simulink model "likestromsmotor"  (R2015a)
settings: Solver=ode45  StartTime=0.0  StopTime=10.0  RelTol=1e-3
values from neighbouring files (symbols this model uses):
  J_m = 0.01    [main.m]
  K_e = K_m    (= 1)    [main.m]
  K_m = 1    [main.m]
  L_a = 1    [main.m]
  M_L = 0    [main.m]
  R_a = 10    [main.m]
  theta_r = pi/2    (= 1.57079632679)    [main.m]
libraries: simulink x1
settings Model: Creator=Martin  LastModifiedBy=Martin

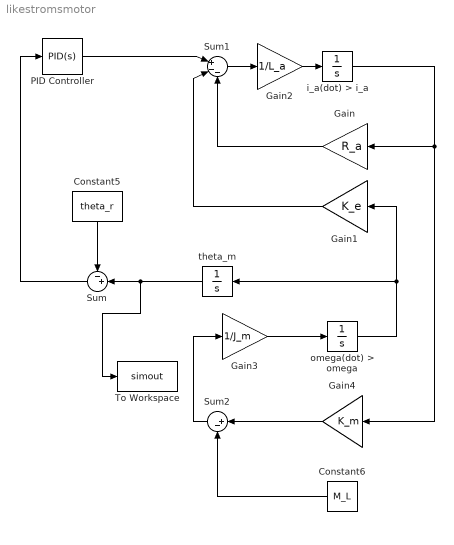
== system likestromsmotor ==
  Constant5 : Constant  Value=theta_r
  Constant6 : Constant  Value=M_L
  Gain : Gain  Gain=R_a
  Gain1 : Gain  Gain=K_e
  Gain2 : Gain  Gain=1/L_a
  Gain3 : Gain  Gain=1/J_m
  Gain4 : Gain  Gain=K_m
  PID Controller : simulink/Continuous/PID Controller  Controller=PID  TimeDomain=Continuous-time  SampleTime=-1  IntegratorMethod=Forward Euler  FilterMethod=Forward Euler  Form=Ideal  UseFilter=on  ControllerParametersSource=internal  P=1  I=0  D=0  N=100  InitialConditionSource=internal  InitialConditionForIntegrator=0  InitialConditionForFilter=0  ExternalReset=none  LimitOutput=off  UpperSaturationLimit=inf  LowerSaturationLimit=-inf  LinearizeAsGain=on  AntiWindupMode=none  Kb=1  TrackingMode=off  Kt=1  PParamMin=[]  PParamMax=[]  IParamMin=[]  IParamMax=[]  DParamMin=[]  DParamMax=[]  NParamMin=[]  NParamMax=[]  KbParamMin=[]  KbParamMax=[]  KtParamMin=[]  KtParamMax=[]  POutMin=[]  POutMax=[]  IOutMin=[]  IOutMax=[]  DOutMin=[]  DOutMax=[]  NOutMin=[]  NOutMax=[]  KbOutMin=[]  KbOutMax=[]  KtOutMin=[]  KtOutMax=[]  IntegratorOutMin=[]  IntegratorOutMax=[]  FilterOutMin=[]  FilterOutMax=[]  SumOutMin=[]  SumOutMax=[]  SumI1OutMin=[]  SumI1OutMax=[]  SumI2OutMin=[]  SumI2OutMax=[]  SumI3OutMin=[]  SumI3OutMax=[]  SumDOutMin=[]  SumDOutMax=[]  SaturationOutMin=[]  SaturationOutMax=[]  IntegratorContinuousStateAttributes=''  IntegratorStateMustResolveToSignalObject=off  IntegratorRTWStateStorageClass=Auto  FilterContinuousStateAttributes=''  FilterStateMustResolveToSignalObject=off  FilterRTWStateStorageClass=Auto  DifferentiatorICPrevScaledInput=0  DifferentiatorOutMin=[]  DifferentiatorOutMax=[]
  Sum : Sum  Inputs=-+|
  Sum1 : Sum  Inputs=|+--
  Sum2 : Sum  Inputs=|+-
  To Workspace : ToWorkspace  VariableName=simout  SaveFormat=Timeseries  SampleTime=-1
  i_a(dot) > i_a : Integrator
  omega(dot) > omega : Integrator
  theta_m : Integrator
  wires:
  Constant5/1 -> Sum/1
  Sum/1 -> PID Controller/1
  PID Controller/1 -> Sum1/1
  i_a(dot) > i_a/1 -> Gain/1, Gain4/1
  Gain/1 -> Sum1/3
  Gain1/1 -> Sum1/2
  Sum1/1 -> Gain2/1
  Gain2/1 -> i_a(dot) > i_a/1
  omega(dot) > omega/1 -> Gain1/1, theta_m/1
  Gain3/1 -> omega(dot) > omega/1
  Gain4/1 -> Sum2/1
  Constant6/1 -> Sum2/2
  Sum2/1 -> Gain3/1
  theta_m/1 -> To Workspace/1, Sum/2
